simulink model "AntiWindup"  (R2020b)
settings: Solver=VariableStepAuto  StartTime=0.0  StopTime=80.0  RelTol=1e-3
settings Model: Creator=lukeb  LastModifiedBy=luke

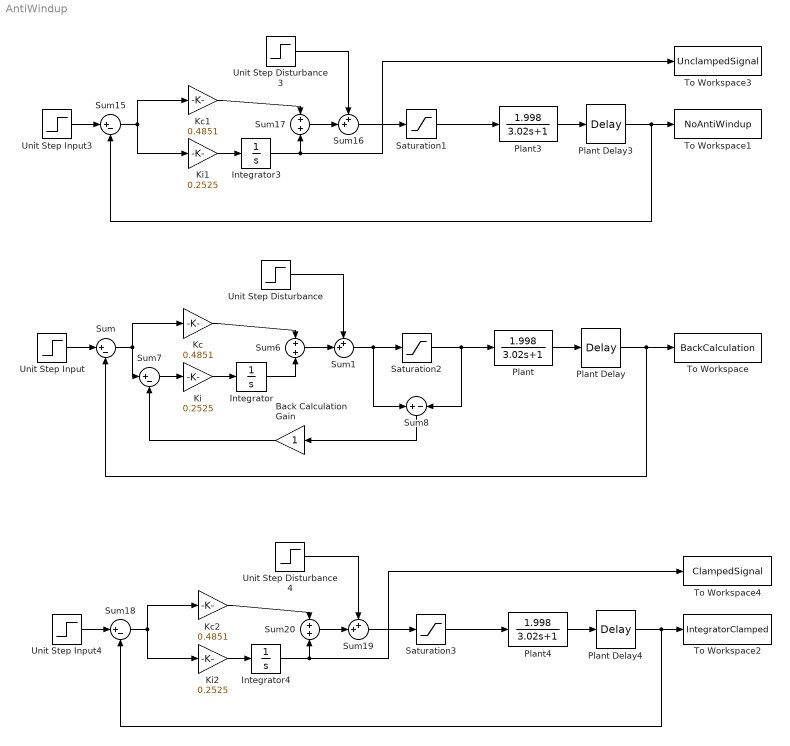
== system AntiWindup ==
  Back Calculation Gain : Gain
  Integrator : Integrator
  Integrator3 : Integrator
  Integrator4 : Integrator  LimitOutput=on  UpperSaturationLimit=0.5  LowerSaturationLimit=-0.5
  Kc : Gain  Gain=0.4851
  Kc1 : Gain  Gain=0.4851
  Kc2 : Gain  Gain=0.4851
  Ki : Gain  Gain=0.2525
  Ki1 : Gain  Gain=0.2525
  Ki2 : Gain  Gain=0.2525
  Plant : TransferFcn  Numerator=[1.998]  Denominator=[3.02 1]
  Plant Delay : TransportDelay  BufferSize=10240
  Plant Delay3 : TransportDelay  BufferSize=10240
  Plant Delay4 : TransportDelay  BufferSize=10240
  Plant3 : TransferFcn  Numerator=[1.998]  Denominator=[3.02 1]
  Plant4 : TransferFcn  Numerator=[1.998]  Denominator=[3.02 1]
  "Saturation1 " : Saturate  UpperLimit=0.75  LowerLimit=-0.75
  Saturation2 : Saturate  UpperLimit=0.75  LowerLimit=-0.75
  Saturation3 : Saturate  UpperLimit=0.75  LowerLimit=-0.75
  Sum{,7,15,18} (4 alike) : Sum  Inputs=|+-
  Sum1 : Sum  Inputs=++|
  Sum16 : Sum  Inputs=++|
  Sum17 : Sum  Inputs=+|+
  Sum19 : Sum  Inputs=++|
  Sum20 : Sum  Inputs=+|+
  Sum6 : Sum  Inputs=+|+
  Sum8 : Sum  Inputs=+|-
  To Workspace : ToWorkspace  VariableName=BackCalculation  SaveFormat=Timeseries  SampleTime=0.0001
  To Workspace1 : ToWorkspace  VariableName=NoAntiWindup  SaveFormat=Timeseries  SampleTime=0.0001
  To Workspace2 : ToWorkspace  VariableName=IntegratorClamped  SaveFormat=Timeseries  SampleTime=0.0001
  To Workspace3 : ToWorkspace  VariableName=UnclampedSignal  SaveFormat=Timeseries  SampleTime=0.0001
  To Workspace4 : ToWorkspace  VariableName=ClampedSignal  SaveFormat=Timeseries  SampleTime=0.0001
  Unit Step Disturbance : Step  Time=40  SampleTime=0
  Unit Step Disturbance3 : Step  Time=40  SampleTime=0
  Unit Step Disturbance4 : Step  Time=40  SampleTime=0
  Unit Step Input : Step  Time=0  SampleTime=0
  Unit Step Input3 : Step  Time=0  SampleTime=0
  Unit Step Input4 : Step  Time=0  SampleTime=0
  wires:
  Sum1/1 -> Saturation2/1, Sum8/1
  Saturation2/1 -> Sum8/2, Plant/1
  Unit Step Disturbance/1 -> Sum1/1
  Unit Step Input/1 -> Sum/1
  Plant Delay/1 -> To Workspace/1, Sum/2
  Plant/1 -> Plant Delay/1
  Sum7/1 -> Ki/1
  Ki/1 -> Integrator/1
  Sum/1 -> Sum7/1, Kc/1
  Integrator/1 -> Sum6/2
  Kc/1 -> Sum6/1
  Sum6/1 -> Sum1/2
  Back Calculation Gain/1 -> Sum7/2
  Sum8/1 -> Back Calculation Gain/1
  Sum15/1 -> Kc1/1, Ki1/1
  Integrator3/1 -> To Workspace3/1, Sum17/2
  Sum17/1 -> Sum16/2
  Sum16/1 -> "Saturation1 "/1
  Plant Delay3/1 -> To Workspace1/1, Sum15/2
  Ki1/1 -> Integrator3/1
  Plant3/1 -> Plant Delay3/1
  Unit Step Input3/1 -> Sum15/1
  "Saturation1 "/1 -> Plant3/1
  Kc1/1 -> Sum17/1
  Unit Step Disturbance3/1 -> Sum16/1
  Unit Step Input4/1 -> Sum18/1
  Plant Delay4/1 -> To Workspace2/1, Sum18/2
  Plant4/1 -> Plant Delay4/1
  Ki2/1 -> Integrator4/1
  Sum19/1 -> Saturation3/1
  Sum18/1 -> Kc2/1, Ki2/1
  Integrator4/1 -> To Workspace4/1, Sum20/2
  Saturation3/1 -> Plant4/1
  Unit Step Disturbance4/1 -> Sum19/1
  Kc2/1 -> Sum20/1
  Sum20/1 -> Sum19/2
